simulink model "if_else_using_junction"  (R2024b)
settings: Solver=VariableStepAuto  StartTime=0.0  StopTime=inf  RelTol=1e-3
settings Model: Creator=rohan  LastModifiedBy=rohan

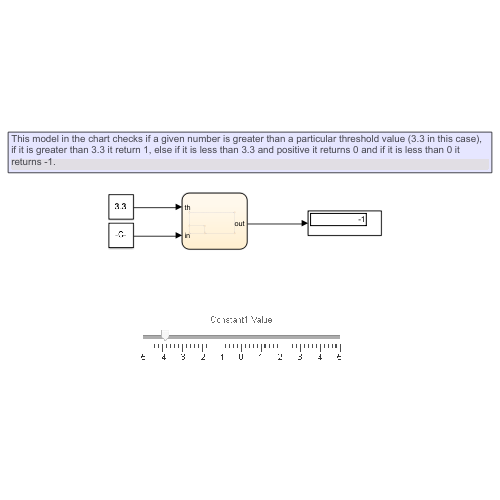
[thumbnail: Simulink's stored preview of the top-level diagram]
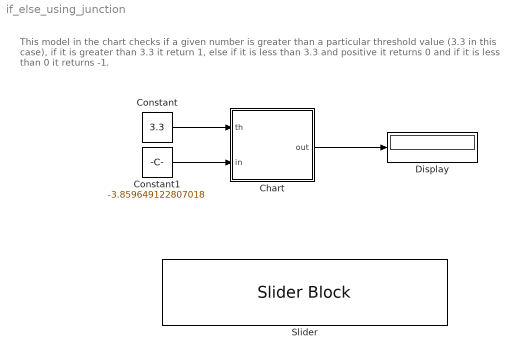
== system if_else_using_junction ==
  note: This model in the chart checks if a given number is greater than a particular threshold value (3.3 in this case),
      | if it is greater than 3.3 it return 1, else if it is less than 3.3 and positive it returns 0 and if it is less than 0 it
      | returns -1.
  Chart : Stateflow chart  TreatAsAtomicUnit=on
  Constant : Constant  Value=3.3
  Constant1 : Constant  Value=-3.859649122807018
  Display : Display
  Slider : SliderBlock  ScaleMin=-5  ScaleMax=5
  wires:
  Constant/1 -> Chart/1(th)
  Constant1/1 -> Chart/2(in)
  Chart/1(out) -> Display/1

== stateflow chart if_else_using_junction/Chart ==
  (default) -> (junction 1)
  (junction 1) -> (junction 3) [order 1] : [in>=th]
  (junction 3) -> (junction 5) : {out=1}
  (junction 1) -> (junction 7) [order 2]
  (junction 7) -> (junction 9) [order 1] : [in<=th&&in>0]
  (junction 7) -> (junction 15) [order 2] : {out=-1}
  (junction 9) -> (junction 12) : {out=0}
  (junction 12) -> (junction 15)
  (junction 5) -> (junction 12)
  data: th input; out output; in input
